simulink model "WithNormalizedLMSFliter"  (R2023b)
settings: Solver=ode3  StartTime=0.0  StopTime=inf  RelTol=1e-3  EnableMultiTasking=on
libraries: raspberrypiAVlib x3, dspsrcs4 x2, dspadpt3 x1
settings Model: FPTRunName=Active  SimulationMode=external  ExtModeTrigDuration=2  Creator=The MathWorks, Inc.  LastModifiedBy=ASUS
settings SolverCC: AlgebraicLoopSolver=TrustRegion  PositivePriorityOrder=on  MaxZcPerStep=1
settings DataIOCC: LimitDataPoints=on  SaveFormat=Array
settings OptimizationCC: ReuseModelBlockBuffer=off  ExpressionDepthLimit=2147483647  LifeSpan=Inf  MaxStackSize=64
settings DebuggingCC: UnderspecifiedInitializationDetection=Classic  MergeDetectMultiDrivingBlocksExec=none  ParameterPrecisionLossMsg=none  FcnCallInpInsideContextMsg=warning  UnconnectedInputMsg=warning  UnconnectedOutputMsg=warning  UnconnectedLineMsg=warning  AllowSymbolicDim=off  StateNameClashWarn=warning  SFUnexpectedBacktrackingDiag=warning  SFNoUnconditionalDefaultTransitionDiag=warning  SFExecutionAtInitializationDiag=none  IntegerSaturationMsg=none  ArithmeticOperatorsInVariantConditions=warning
settings HardwareCC: ProdBitPerPointer=32  ProdBitPerSizeT=32  ProdBitPerPtrDiffT=32  ProdLargestAtomicInteger=Long  ProdLargestAtomicFloat=Double  ProdWordSize=32  ProdHWDeviceType=ARM Compatible->ARM Cortex  UseEmbeddedCoderFeatures=off  UseSimulinkCoderFeatures=off
settings ModelReferenceCC: EnableRefExpFcnMdlSchedulingChecks=on  PropagateSignalLabelsOutOfModel=off
settings SFSimCC: SimUseLocalCustomCode=off  CustomCodeUndefinedFunction=UseInterfaceOnly
settings RTWCC: Description=Embedded Coder  SystemTargetFile=ert.tlc  HardwareBoard=Raspberry Pi  TemplateMakefile=ert_default_tmf  RTWVerbose=off  RTWUseLocalCustomCode=off  Toolchain=GNU GCC Embedded Linux  BuildConfiguration=Faster Runs  DLArmComputeVersion=19.05
settings CodeAppCC: ForceParamTrailComments=on  OperatorAnnotations=on  MangleLength=10  StateflowObjectComments=on  MATLABSourceComments=on
settings ERTTargetCC: MultiwordLength=2048  ERTCustomFileBanners=off  SupportContinuousTime=on  SupportNonInlinedSFcns=on  RemoveResetFunc=off  SupportVariableSizeSignals=on  ModelStepFunctionPrototypeControlCompliant=off  ExtMode=on  ExtModeTransport=2  ExtModeStaticAlloc=on  ExtModeMaxTrigDuration=1000  ExtModeMexFile=ext_xcp  ExtModeMexArgs='192.168.127.146' 0 17725  ExtModeIntrfLevel=Level2 - Open  ERTSrcFileBannerTemplate=codertarget_code_template.cgt  ERTHdrFileBannerTemplate=codertarget_code_template.cgt  ERTDataSrcFileTemplate=codertarget_code_template.cgt  ERTDataHdrFileTemplate=codertarget_code_template.cgt
settings ConfigComp: CovMetricSettings=dw  CovSaveCumulativeToWorkspaceVar=on  CovSaveSingleToWorkspaceVar=on  CovExternalEMLEnable=off  CovSFcnEnable=off

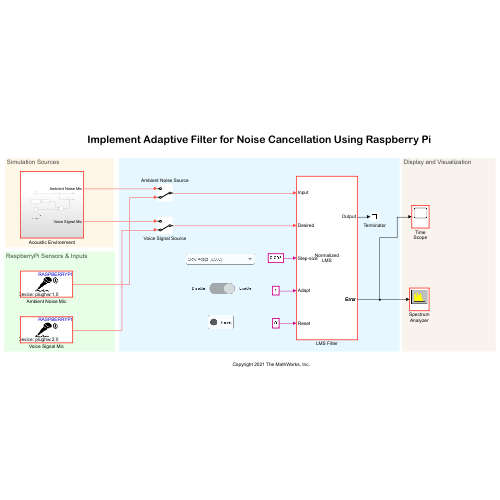
[thumbnail: Simulink's stored preview of the top-level diagram]
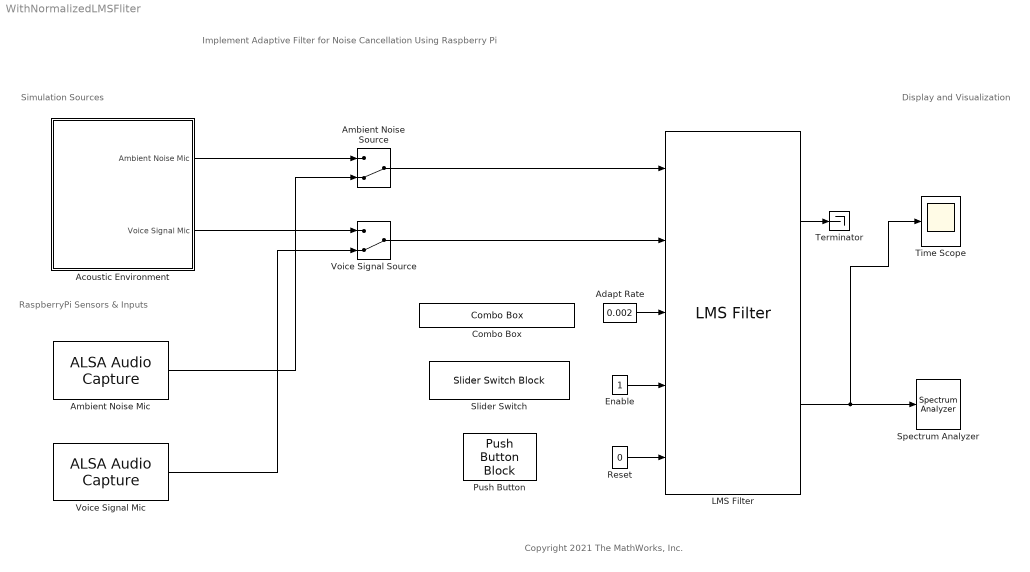
== system WithNormalizedLMSFliter ==
  note: Simulation Sources
  note: Display and Visualization
  note: Implement Adaptive Filter for Noise Cancellation Using Raspberry Pi
  note: RaspberryPi Sensors & Inputs
  note: Copyright 2021 The MathWorks, Inc.
  Acoustic Environment : Subsystem
  Adapt Rate : Constant  Value=0.002  OutDataTypeStr=single
  Ambient Noise Mic : raspberrypiAVlib/ALSA Audio Capture  deviceStr='plughw:1,0'  DataBitDepth=16-bit integer  numberOfChannels=1  sampleRateEnum=8000  frameSize=800  QueueDuration=0.5  blockPlatform=Raspberry Pi
  Ambient Noise Source : ManualSwitch  CurrentSetting=0
  Combo Box : ComboBox  LabelPosition=Hide  SelectedLabel=Slow Adapt (0.002)
      settings: Values={{'Slow Adapt (0.002)', 'Medium Adapt (0.01)', 'Fast Adapt (0.04)'}, [0.002 0.01 0.04]}
  Enable : Constant  OutDataTypeStr=boolean
  LMS Filter : dspadpt3/LMS Filter  Algo=Normalized LMS  L=40  stepflag=Input port  mu=0.1  leakage=1.0  ic=0  Adapt=on  resetflag=Non-zero sample  weights=off  addnparflag=off  roundingMode=Floor  overflowMode=off  secondCoeffMode=Binary point scaling  secondCoeffWordLength=2  secondCoeffFracLength=15  prodOutput2Mode=Binary point scaling  prodOutput2FracLength=20  prodOutput3Mode=Binary point scaling  prodOutput3FracLength=20  prodOutput4Mode=Binary point scaling  prodOutput4FracLength=20  quotientMode=Binary point scaling  quotientFracLength=20  accum2Mode=Binary point scaling  accum2FracLength=20
  Push Button : PushButtonBlock  ButtonText=Reset  Icon=Circle  OffValue=0.000000
  Reset : Constant  Value=0  OutDataTypeStr=boolean
  Slider Switch : SliderSwitchBlock  LabelPosition=Hide
      settings: Values={{'Disable', 'Enable'}, [0 1]}
  Spectrum Analyzer : SpectrumAnalyzer  WindowPosition=[780.000000,175.000000,513.000000,432.000000,]  ScopeFrameLocation=window  SampleRateSource=Property  SampleRate=44.1e3  PlotAsTwoSidedSpectrum=off  AveragingMethod=Exponential  YLimits=[-44.33479165,8.94078475]
      settings: OpenAtSimulationStart=off
  Terminator : Terminator
  Time Scope : Scope
  Voice Signal Mic : raspberrypiAVlib/ALSA Audio Capture  deviceStr='plughw:2,0'  DataBitDepth=16-bit integer  numberOfChannels=1  sampleRateEnum=8000  frameSize=800  QueueDuration=0.5  blockPlatform=Raspberry Pi
  Voice Signal Source : ManualSwitch  CurrentSetting=0
  wires:
  Acoustic Environment/1(Ambient Noise Mic) -> Ambient Noise Source/1
  Ambient Noise Mic/1 -> Ambient Noise Source/2
  Acoustic Environment/2(Voice Signal Mic) -> Voice Signal Source/1
  Voice Signal Mic/1 -> Voice Signal Source/2
  Ambient Noise Source/1 -> LMS Filter/1
  Voice Signal Source/1 -> LMS Filter/2
  Reset/1 -> LMS Filter/5
  Enable/1 -> LMS Filter/4
  Adapt Rate/1 -> LMS Filter/3
  LMS Filter/1 -> Terminator/1
  LMS Filter/2 -> Time Scope/1, Spectrum Analyzer/1

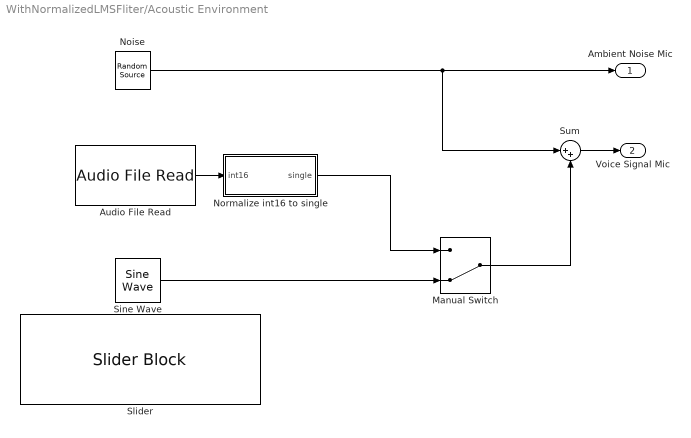
== system WithNormalizedLMSFliter/Acoustic Environment ==
  Audio File Read : raspberrypiAVlib/Audio File Read  FileName=dspafxf_8000.wav  PlayCount=Inf  OutputEOFIndicator=off  SamplesPerFrame=800
  Manual Switch : ManualSwitch  CurrentSetting=0
  Noise : dspsrcs4/Random Source  SrcType=Gaussian  NormMethod=Sum of uniform values  CltLength=5  MinVal=-1  MaxVal=1  MeanVal=0  VarVal=1  RepMode=Specify seed  rawSeed=[23341]  IsInherit=off  SampMode=Discrete  SampTime=1/8000  SampFrame=800  DataType=Single  OutComplex=Real  OutputFrames=off
  Normalize int16 to single : Subsystem
  Sine Wave : dspsrcs4/Sine Wave  Amplitude=1  Frequency=868.6743079584775  Phase=0  SampleMode=Discrete  OutComplex=Real  CompMethod=Trigonometric fcn  TableSize=Speed  SampleTime=1/8000  SamplesPerFrame=800  ResetState=Restart at time zero  OutputFrames=off  dataType=single  wordLen=16  udDataType=sfix(16)  fracBitsMode=Best precision  numFracBits=15  OutDataTypeStr=single  LastOutDataTypeStr=single
  Slider : SliderBlock  LabelPosition=Bottom  ScaleMin=500  ScaleMax=1000  TickInterval=100
  Sum : Sum  Inputs=|++  InputSameDT=on  SaturateOnIntegerOverflow=on  OutDataTypeStr=Inherit: Same as first input
  Ambient Noise Mic : Outport
  Voice Signal Mic : Outport  Port=2
  wires:
  Sum/1 -> Voice Signal Mic/1
  Noise/1 -> Ambient Noise Mic/1, Sum/1
  Audio File Read/1 -> Normalize int16 to single/1(int16)
  Manual Switch/1 -> Sum/2
  Normalize int16 to single/1(single) -> Manual Switch/1
  Sine Wave/1 -> Manual Switch/2

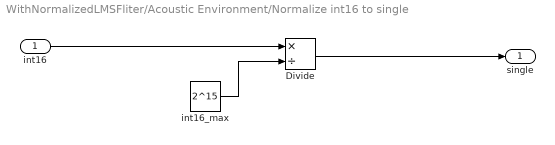
== system WithNormalizedLMSFliter/Acoustic Environment/Normalize int16 to single ==
  int16 : Inport
  Divide : Product  Inputs=*/  OutDataTypeStr=single
  int16_max : Constant  Value=2^15  OutDataTypeStr=single  SampleTime=-1
  single : Outport
  wires:
  int16_max/1 -> Divide/2
  Divide/1 -> single/1
  int16/1 -> Divide/1
